simulink model "openWaterModel"  (R2020a)
settings: Solver=FixedStepAuto  StartTime=0.0  StopTime=inf  FixedStep=Ts  RelTol=1e-3  EnableMultiTasking=on
values from neighbouring files (symbols this model uses):
  ctrlMap =     [init_Kite.mat]
  Ts = 0.01    [init_Kite.mat]
undefined symbols (not defined in the file or in its folder): initializeBussesFromBlock, IO397, standard
libraries: xpcutilitieslib x172, hdlsllib x100, simulink x36, dspsigops x13, slrtlib x4, xpcseriallib x3, speedgoatlib_fpga_analog_io x2, xpcrtudplib x2, speedgoatlib_fpga_dio x1, speedgoatlib_fpga_quadrature x1, speedgoatlib_IO581 x1, speedgoatlib_fpga x1
(part 3 of 4)

== system openWaterModel/Sensor Processing/IMU Processing/Controller1/FilteredPIDController2 ==
  note: Tau with minimum
  note: Anti-winding
  del_u : Inport
  Abs : Abs
  Add1 : Sum  Inputs=+++
  Add2 : Sum  Inputs=+-
  Constant : Constant
  Constant1 : Constant  Value=0
  Constant2 : Constant
  Divide{1..4} (4 alike) : Product  Inputs=*/
  Int_reset : Constant  Value=0
  Integrator : Integrator
  Integrator3 : Integrator  ExternalReset=either
  Max : MinMax  Function=max  Inputs=2
  Product : Product
  Product1 : Product
  RollKd : Gain
  RollKi : Gain  Gain=0
  RollKp : Gain  Gain=3
  RollTau : Constant  Value=0.02
  Switch : Switch  Threshold=30
  Weighted Sample Time : SampleTimeMath  TsampMathOp=Ts Only
  const : Constant
  y : Outport
  wires:
  Product1/1 -> Divide2/1
  [stop_trig] -> Product1/1
  RollKi/1 -> Product1/2
  Switch/1 -> [stop_trig]
  Constant2/1 -> Switch/3
  Constant1/1 -> Switch/1
  Abs/1 -> Switch/2
  [y] -> Abs/1
  Add2/1 -> Integrator/1, Product/2
  Divide4/1 -> Add2/2
  del_u/1 -> Add2/1
  [Tau] -> Divide4/2
  [Tau] -> Divide3/2
  Divide3/1 -> Add1/3
  RollKp/1 -> Divide3/1
  Product/1 -> Add1/1
  Integrator3/1 -> Add1/2
  Divide2/1 -> Integrator3/1
  [Tau] -> Divide2/2
  Integrator/1 -> RollKi/1, Divide4/1, RollKp/1
  Divide1/1 -> Product/1
  [Tau] -> Divide1/2
  Constant/1 -> RollKd/1
  RollKd/1 -> Divide1/1
  Max/1 -> [Tau]
  Weighted Sample Time/1 -> Max/1
  const/1 -> Weighted Sample Time/1
  Add1/1 -> y/1, [y]
  RollTau/1 -> Max/2
  Int_reset/1 -> Integrator3/2

== system openWaterModel/Sensor Processing/IMU Processing/Controller1/FilteredPIDController_Pitchold ==
  del_u : Inport
  Add : Sum  Inputs=+-
  Add1 : Sum  Inputs=+++
  Divide : Product  Inputs=*/
  Integrator : Integrator
  Integrator1 : Integrator
  Integrator2 : Integrator
  Max : MinMax  Function=max  Inputs=2
  PitchKd : Gain
  PitchKi : Gain  Gain=0
  PitchKp : Gain
  PitchTau : Constant  Value=0.1
  Weighted Sample Time : SampleTimeMath  TsampMathOp=Ts Only
  const : Constant
  y : Outport
  wires:
  PitchTau/1 -> Max/2
  Divide/1 -> y/1, [y]
  Add/1 -> Integrator/1
  const/1 -> Weighted Sample Time/1
  Integrator/1 -> Add1/1
  Integrator1/1 -> Integrator2/1
  [y] -> Add/2
  Max/1 -> Divide/2
  PitchKd/1 -> Add1/3
  Add1/1 -> Divide/1
  PitchKi/1 -> Integrator1/1
  PitchKp/1 -> Add/1
  Weighted Sample Time/1 -> Max/1
  Integrator2/1 -> Add1/2
  del_u/1 -> PitchKd/1, PitchKi/1, PitchKp/1

== system openWaterModel/Sensor Processing/IMU Processing/Controller1/FilteredPIDController_oldRoll ==
  del_u : Inport
  Add : Sum  Inputs=+-
  Add1 : Sum  Inputs=+++
  Divide : Product  Inputs=*/
  Integrator : Integrator
  Integrator1 : Integrator
  Integrator2 : Integrator
  Max : MinMax  Function=max  Inputs=2
  RollKd : Gain
  RollKi : Gain  Gain=0
  RollKp : Gain
  RollTau : Constant  Value=0.1
  Weighted Sample Time : SampleTimeMath  TsampMathOp=Ts Only
  const : Constant
  y : Outport
  wires:
  RollTau/1 -> Max/2
  Divide/1 -> y/1, [y]
  Add/1 -> Integrator/1
  const/1 -> Weighted Sample Time/1
  Integrator/1 -> Add1/1
  Integrator1/1 -> Integrator2/1
  [y] -> Add/2
  Max/1 -> Divide/2
  RollKd/1 -> Add1/3
  Add1/1 -> Divide/1
  RollKi/1 -> Integrator1/1
  RollKp/1 -> Add/1
  Weighted Sample Time/1 -> Max/1
  Integrator2/1 -> Add1/2
  del_u/1 -> RollKd/1, RollKi/1, RollKp/1

== system openWaterModel/Sensor Processing/IMU Processing/Controller1/FilteredPIDController_oldYaw ==
  del_u : Inport
  Add : Sum  Inputs=+-
  Add1 : Sum  Inputs=+++
  Divide : Product  Inputs=*/
  Integrator : Integrator
  Integrator1 : Integrator
  Integrator2 : Integrator
  Max : MinMax  Function=max  Inputs=2
  Weighted Sample Time : SampleTimeMath  TsampMathOp=Ts Only
  YawKd : Gain  Gain=0.2
  YawKi : Gain  Gain=0.3
  YawKp : Gain  Gain=0.1
  YawTau : Constant  Value=0.4
  const : Constant
  y : Outport
  wires:
  YawTau/1 -> Max/2
  Divide/1 -> y/1, [y]
  Add/1 -> Integrator/1
  const/1 -> Weighted Sample Time/1
  Integrator/1 -> Add1/1
  Integrator1/1 -> Integrator2/1
  [y] -> Add/2
  Max/1 -> Divide/2
  YawKd/1 -> Add1/3
  Add1/1 -> Divide/1
  YawKi/1 -> Integrator1/1
  YawKp/1 -> Add/1
  Weighted Sample Time/1 -> Max/1
  Integrator2/1 -> Add1/2
  del_u/1 -> YawKd/1, YawKi/1, YawKp/1

== system openWaterModel/Sensor Processing/IMU Processing/Kite Measurements /Enabled Subsystem ==
  Double : Inport
  Enable : EnablePort
  Out1 : Outport
  wires:
  Double/1 -> Out1/1

== system openWaterModel/Sensor Processing/IMU Processing/Kite Measurements /Enabled Subsystem1 ==
  Double : Inport
  Enable : EnablePort
  Out1 : Outport
  wires:
  Double/1 -> Out1/1

== system openWaterModel/Sensor Processing/IMU Processing/Kite Measurements /Enabled Subsystem10 ==
  Double : Inport
  Enable : EnablePort
  Out1 : Outport
  wires:
  Double/1 -> Out1/1

== system openWaterModel/Sensor Processing/IMU Processing/Kite Measurements /Enabled Subsystem11 ==
  Double : Inport
  Enable : EnablePort
  Out1 : Outport
  wires:
  Double/1 -> Out1/1

== system openWaterModel/Sensor Processing/IMU Processing/Kite Measurements /Enabled Subsystem12 ==
  Double : Inport
  Enable : EnablePort
  Out1 : Outport
  wires:
  Double/1 -> Out1/1

== system openWaterModel/Sensor Processing/IMU Processing/Kite Measurements /Enabled Subsystem13 ==
  Double : Inport
  Enable : EnablePort
  Out1 : Outport
  wires:
  Double/1 -> Out1/1

== system openWaterModel/Sensor Processing/IMU Processing/Kite Measurements /Enabled Subsystem14 ==
  Double : Inport
  Enable : EnablePort
  Out1 : Outport
  wires:
  Double/1 -> Out1/1

== system openWaterModel/Sensor Processing/IMU Processing/Kite Measurements /Enabled Subsystem15 ==
  Double : Inport
  Enable : EnablePort
  Out1 : Outport
  wires:
  Double/1 -> Out1/1

== system openWaterModel/Sensor Processing/IMU Processing/Kite Measurements /Enabled Subsystem16 ==
  Double : Inport
  Enable : EnablePort
  Out1 : Outport
  wires:
  Double/1 -> Out1/1

== system openWaterModel/Sensor Processing/IMU Processing/Kite Measurements /Enabled Subsystem17 ==
  Double : Inport
  Enable : EnablePort
  Out1 : Outport
  wires:
  Double/1 -> Out1/1

== system openWaterModel/Sensor Processing/IMU Processing/Kite Measurements /Enabled Subsystem18 ==
  Double : Inport
  Enable : EnablePort
  Out1 : Outport
  wires:
  Double/1 -> Out1/1

== system openWaterModel/Sensor Processing/IMU Processing/Kite Measurements /Enabled Subsystem19 ==
  Double : Inport
  Enable : EnablePort
  Out1 : Outport
  wires:
  Double/1 -> Out1/1

== system openWaterModel/Sensor Processing/IMU Processing/Kite Measurements /Enabled Subsystem2 ==
  Double : Inport
  Enable : EnablePort
  Out1 : Outport
  wires:
  Double/1 -> Out1/1

== system openWaterModel/Sensor Processing/IMU Processing/Kite Measurements /Enabled Subsystem3 ==
  Double : Inport
  Enable : EnablePort
  Out1 : Outport
  wires:
  Double/1 -> Out1/1

== system openWaterModel/Sensor Processing/IMU Processing/Kite Measurements /Enabled Subsystem4 ==
  Double : Inport
  Enable : EnablePort
  Out1 : Outport
  wires:
  Double/1 -> Out1/1

== system openWaterModel/Sensor Processing/IMU Processing/Kite Measurements /Enabled Subsystem5 ==
  Double : Inport
  Enable : EnablePort
  Out1 : Outport
  wires:
  Double/1 -> Out1/1

== system openWaterModel/Sensor Processing/IMU Processing/Kite Measurements /Enabled Subsystem6 ==
  Double : Inport
  Enable : EnablePort
  Out1 : Outport
  wires:
  Double/1 -> Out1/1

== system openWaterModel/Sensor Processing/IMU Processing/Kite Measurements /Enabled Subsystem7 ==
  Double : Inport
  Enable : EnablePort
  Out1 : Outport
  wires:
  Double/1 -> Out1/1

== system openWaterModel/Sensor Processing/IMU Processing/Kite Measurements /Enabled Subsystem8 ==
  Double : Inport
  Enable : EnablePort
  Out1 : Outport
  wires:
  Double/1 -> Out1/1

== system openWaterModel/Sensor Processing/IMU Processing/Kite Measurements /Enabled Subsystem9 ==
  Double : Inport
  Enable : EnablePort
  Out1 : Outport
  wires:
  Double/1 -> Out1/1

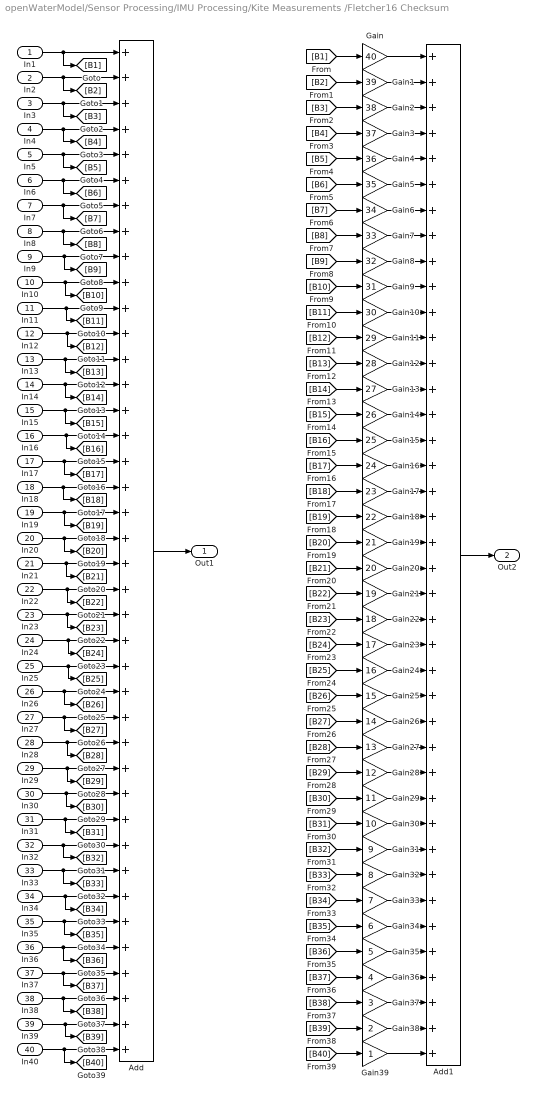
== system openWaterModel/Sensor Processing/IMU Processing/Kite Measurements /Fletcher16 Checksum ==
  In1 : Inport
  In2 : Inport  Port=2
  In3 : Inport  Port=3
  In4 : Inport  Port=4
  In5 : Inport  Port=5
  In6 : Inport  Port=6
  In7 : Inport  Port=7
  In8 : Inport  Port=8
  In9 : Inport  Port=9
  In10 : Inport  Port=10
  In11 : Inport  Port=11
  In12 : Inport  Port=12
  In13 : Inport  Port=13
  In14 : Inport  Port=14
  In15 : Inport  Port=15
  In16 : Inport  Port=16
  In17 : Inport  Port=17
  In18 : Inport  Port=18
  In19 : Inport  Port=19
  In20 : Inport  Port=20
  In21 : Inport  Port=21
  In22 : Inport  Port=22
  In23 : Inport  Port=23
  In24 : Inport  Port=24
  In25 : Inport  Port=25
  In26 : Inport  Port=26
  In27 : Inport  Port=27
  In28 : Inport  Port=28
  In29 : Inport  Port=29
  In30 : Inport  Port=30
  In31 : Inport  Port=31
  In32 : Inport  Port=32
  In33 : Inport  Port=33
  In34 : Inport  Port=34
  In35 : Inport  Port=35
  In36 : Inport  Port=36
  In37 : Inport  Port=37
  In38 : Inport  Port=38
  In39 : Inport  Port=39
  In40 : Inport  Port=40
  Add : Sum  Inputs=++++++++++++++++++++++++++++++++++++++++
  Add1 : Sum  Inputs=++++++++++++++++++++++++++++++++++++++++
  Gain : Gain  Gain=40  OutDataTypeStr=uint8
  Gain1 : Gain  Gain=39  OutDataTypeStr=uint8
  Gain10 : Gain  Gain=30  OutDataTypeStr=uint8
  Gain11 : Gain  Gain=29  OutDataTypeStr=uint8
  Gain12 : Gain  Gain=28  OutDataTypeStr=uint8
  Gain13 : Gain  Gain=27  OutDataTypeStr=uint8
  Gain14 : Gain  Gain=26  OutDataTypeStr=uint8
  Gain15 : Gain  Gain=25  OutDataTypeStr=uint8
  Gain16 : Gain  Gain=24  OutDataTypeStr=uint8
  Gain17 : Gain  Gain=23  OutDataTypeStr=uint8
  Gain18 : Gain  Gain=22  OutDataTypeStr=uint8
  Gain19 : Gain  Gain=21  OutDataTypeStr=uint8
  Gain2 : Gain  Gain=38  OutDataTypeStr=uint8
  Gain20 : Gain  Gain=20  OutDataTypeStr=uint8
  Gain21 : Gain  Gain=19  OutDataTypeStr=uint8
  Gain22 : Gain  Gain=18  OutDataTypeStr=uint8
  Gain23 : Gain  Gain=17  OutDataTypeStr=uint8
  Gain24 : Gain  Gain=16  OutDataTypeStr=uint8
  Gain25 : Gain  Gain=15  OutDataTypeStr=uint8
  Gain26 : Gain  Gain=14  OutDataTypeStr=uint8
  Gain27 : Gain  Gain=13  OutDataTypeStr=uint8
  Gain28 : Gain  Gain=12  OutDataTypeStr=uint8
  Gain29 : Gain  Gain=11  OutDataTypeStr=uint8
  Gain3 : Gain  Gain=37  OutDataTypeStr=uint8
  Gain30 : Gain  Gain=10  OutDataTypeStr=uint8
  Gain31 : Gain  Gain=9  OutDataTypeStr=uint8
  Gain32 : Gain  Gain=8  OutDataTypeStr=uint8
  Gain33 : Gain  Gain=7  OutDataTypeStr=uint8
  Gain34 : Gain  Gain=6  OutDataTypeStr=uint8
  Gain35 : Gain  Gain=5  OutDataTypeStr=uint8
  Gain36 : Gain  Gain=4  OutDataTypeStr=uint8
  Gain37 : Gain  Gain=3  OutDataTypeStr=uint8
  Gain38 : Gain  Gain=2  OutDataTypeStr=uint8
  Gain39 : Gain  OutDataTypeStr=uint8
  Gain4 : Gain  Gain=36  OutDataTypeStr=uint8
  Gain5 : Gain  Gain=35  OutDataTypeStr=uint8
  Gain6 : Gain  Gain=34  OutDataTypeStr=uint8
  Gain7 : Gain  Gain=33  OutDataTypeStr=uint8
  Gain8 : Gain  Gain=32  OutDataTypeStr=uint8
  Gain9 : Gain  Gain=31  OutDataTypeStr=uint8
  Out1 : Outport
  Out2 : Outport  Port=2
  wires:
  In3/1 -> [B3], Add/3
  [B4] -> Gain3/1
  In2/1 -> [B2], Add/2
  [B1] -> Gain/1
  Add1/1 -> Out2/1
  In4/1 -> [B4], Add/4
  [B3] -> Gain2/1
  In6/1 -> [B6], Add/6
  In5/1 -> [B5], Add/5
  [B2] -> Gain1/1
  [B5] -> Gain4/1
  In1/1 -> Add/1, [B1]
  Add/1 -> Out1/1
  In7/1 -> [B7], Add/7
  In8/1 -> [B8], Add/8
  In9/1 -> [B9], Add/9
  In10/1 -> [B10], Add/10
  In11/1 -> [B11], Add/11
  In12/1 -> [B12], Add/12
  In13/1 -> [B13], Add/13
  In14/1 -> [B14], Add/14
  In15/1 -> [B15], Add/15
  In16/1 -> [B16], Add/16
  In17/1 -> [B17], Add/17
  In18/1 -> [B18], Add/18
  In19/1 -> [B19], Add/19
  In20/1 -> [B20], Add/20
  In21/1 -> [B21], Add/21
  In22/1 -> [B22], Add/22
  In23/1 -> [B23], Add/23
  In24/1 -> [B24], Add/24
  In25/1 -> [B25], Add/25
  In26/1 -> [B26], Add/26
  In27/1 -> [B27], Add/27
  In28/1 -> [B28], Add/28
  In29/1 -> [B29], Add/29
  In30/1 -> [B30], Add/30
  In31/1 -> [B31], Add/31
  In32/1 -> [B32], Add/32
  In33/1 -> [B33], Add/33
  In34/1 -> [B34], Add/34
  In35/1 -> [B35], Add/35
  In36/1 -> [B36], Add/36
  In37/1 -> [B37], Add/37
  In38/1 -> [B38], Add/38
  In39/1 -> [B39], Add/39
  In40/1 -> [B40], Add/40
  Gain/1 -> Add1/1
  Gain1/1 -> Add1/2
  Gain2/1 -> Add1/3
  Gain3/1 -> Add1/4
  Gain4/1 -> Add1/5
  [B6] -> Gain5/1
  Gain5/1 -> Add1/6
  [B7] -> Gain6/1
  Gain6/1 -> Add1/7
  Gain7/1 -> Add1/8
  [B8] -> Gain7/1
  [B9] -> Gain8/1
  Gain8/1 -> Add1/9
  Gain9/1 -> Add1/10
  [B10] -> Gain9/1
  [B11] -> Gain10/1
  Gain10/1 -> Add1/11
  [B12] -> Gain11/1
  [B13] -> Gain12/1
  [B14] -> Gain13/1
  Gain13/1 -> Add1/14
  [B15] -> Gain14/1
  Gain14/1 -> Add1/15
  [B16] -> Gain15/1
  Gain15/1 -> Add1/16
  [B17] -> Gain16/1
  Gain16/1 -> Add1/17
  [B18] -> Gain17/1
  Gain17/1 -> Add1/18
  [B19] -> Gain18/1
  Gain18/1 -> Add1/19
  [B20] -> Gain19/1
  Gain19/1 -> Add1/20
  [B21] -> Gain20/1
  Gain20/1 -> Add1/21
  [B22] -> Gain21/1
  Gain21/1 -> Add1/22
  [B23] -> Gain22/1
  Gain22/1 -> Add1/23
  [B24] -> Gain23/1
  Gain23/1 -> Add1/24
  [B25] -> Gain24/1
  Gain24/1 -> Add1/25
  [B26] -> Gain25/1
  Gain25/1 -> Add1/26
  [B27] -> Gain26/1
  Gain26/1 -> Add1/27
  [B28] -> Gain27/1
  Gain27/1 -> Add1/28
  [B29] -> Gain28/1
  Gain28/1 -> Add1/29
  [B30] -> Gain29/1
  Gain29/1 -> Add1/30
  [B31] -> Gain30/1
  Gain30/1 -> Add1/31
  [B32] -> Gain31/1
  Gain31/1 -> Add1/32
  [B33] -> Gain32/1
  Gain32/1 -> Add1/33
  [B34] -> Gain33/1
  Gain33/1 -> Add1/34
  [B35] -> Gain34/1
  Gain34/1 -> Add1/35
  [B36] -> Gain35/1
  Gain35/1 -> Add1/36
  [B37] -> Gain36/1
  Gain36/1 -> Add1/37
  [B38] -> Gain37/1
  Gain37/1 -> Add1/38
  [B39] -> Gain38/1
  Gain38/1 -> Add1/39
  [B40] -> Gain39/1
  Gain39/1 -> Add1/40
  Gain11/1 -> Add1/12
  Gain12/1 -> Add1/13

== system openWaterModel/Sensor Processing/IMU Processing/Kite Measurements /Fletcher16 Checksum1 ==
  In1 : Inport
  In2 : Inport  Port=2
  In3 : Inport  Port=3
  In4 : Inport  Port=4
  Add : Sum  Inputs=4
  Add1 : Sum  Inputs=++++
  Gain : Gain  Gain=4  OutDataTypeStr=uint8
  Gain1 : Gain  Gain=3  OutDataTypeStr=uint8
  Gain2 : Gain  Gain=2  OutDataTypeStr=uint8
  Gain3 : Gain  OutDataTypeStr=uint8
  Out1 : Outport
  Out2 : Outport  Port=2
  wires:
  Gain3/1 -> Add1/4
  Gain2/1 -> Add1/3
  Gain1/1 -> Add1/2
  Gain/1 -> Add1/1
  Add/1 -> Out1/1
  In1/1 -> [B1], Add/1
  [B2] -> Gain1/1
  [B3] -> Gain2/1
  In4/1 -> [B4], Add/4
  Add1/1 -> Out2/1
  [B1] -> Gain/1
  In2/1 -> [B2], Add/2
  [B4] -> Gain3/1
  In3/1 -> [B3], Add/3

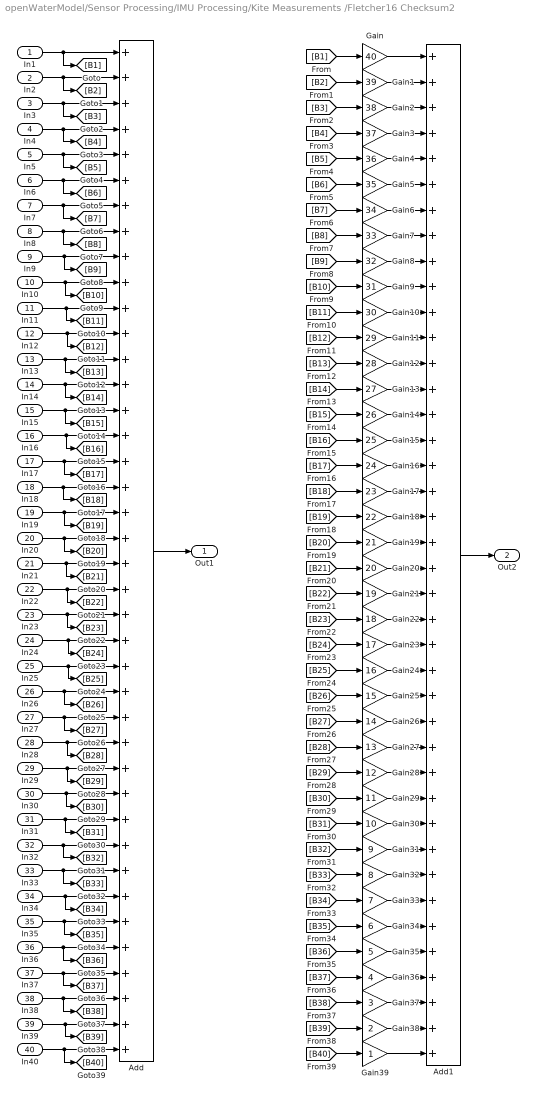
== system openWaterModel/Sensor Processing/IMU Processing/Kite Measurements /Fletcher16 Checksum2 ==
  In1 : Inport
  In2 : Inport  Port=2
  In3 : Inport  Port=3
  In4 : Inport  Port=4
  In5 : Inport  Port=5
  In6 : Inport  Port=6
  In7 : Inport  Port=7
  In8 : Inport  Port=8
  In9 : Inport  Port=9
  In10 : Inport  Port=10
  In11 : Inport  Port=11
  In12 : Inport  Port=12
  In13 : Inport  Port=13
  In14 : Inport  Port=14
  In15 : Inport  Port=15
  In16 : Inport  Port=16
  In17 : Inport  Port=17
  In18 : Inport  Port=18
  In19 : Inport  Port=19
  In20 : Inport  Port=20
  In21 : Inport  Port=21
  In22 : Inport  Port=22
  In23 : Inport  Port=23
  In24 : Inport  Port=24
  In25 : Inport  Port=25
  In26 : Inport  Port=26
  In27 : Inport  Port=27
  In28 : Inport  Port=28
  In29 : Inport  Port=29
  In30 : Inport  Port=30
  In31 : Inport  Port=31
  In32 : Inport  Port=32
  In33 : Inport  Port=33
  In34 : Inport  Port=34
  In35 : Inport  Port=35
  In36 : Inport  Port=36
  In37 : Inport  Port=37
  In38 : Inport  Port=38
  In39 : Inport  Port=39
  In40 : Inport  Port=40
  Add : Sum  Inputs=++++++++++++++++++++++++++++++++++++++++
  Add1 : Sum  Inputs=++++++++++++++++++++++++++++++++++++++++
  Gain : Gain  Gain=40  OutDataTypeStr=uint8
  Gain1 : Gain  Gain=39  OutDataTypeStr=uint8
  Gain10 : Gain  Gain=30  OutDataTypeStr=uint8
  Gain11 : Gain  Gain=29  OutDataTypeStr=uint8
  Gain12 : Gain  Gain=28  OutDataTypeStr=uint8
  Gain13 : Gain  Gain=27  OutDataTypeStr=uint8
  Gain14 : Gain  Gain=26  OutDataTypeStr=uint8
  Gain15 : Gain  Gain=25  OutDataTypeStr=uint8
  Gain16 : Gain  Gain=24  OutDataTypeStr=uint8
  Gain17 : Gain  Gain=23  OutDataTypeStr=uint8
  Gain18 : Gain  Gain=22  OutDataTypeStr=uint8
  Gain19 : Gain  Gain=21  OutDataTypeStr=uint8
  Gain2 : Gain  Gain=38  OutDataTypeStr=uint8
  Gain20 : Gain  Gain=20  OutDataTypeStr=uint8
  Gain21 : Gain  Gain=19  OutDataTypeStr=uint8
  Gain22 : Gain  Gain=18  OutDataTypeStr=uint8
  Gain23 : Gain  Gain=17  OutDataTypeStr=uint8
  Gain24 : Gain  Gain=16  OutDataTypeStr=uint8
  Gain25 : Gain  Gain=15  OutDataTypeStr=uint8
  Gain26 : Gain  Gain=14  OutDataTypeStr=uint8
  Gain27 : Gain  Gain=13  OutDataTypeStr=uint8
  Gain28 : Gain  Gain=12  OutDataTypeStr=uint8
  Gain29 : Gain  Gain=11  OutDataTypeStr=uint8
  Gain3 : Gain  Gain=37  OutDataTypeStr=uint8
  Gain30 : Gain  Gain=10  OutDataTypeStr=uint8
  Gain31 : Gain  Gain=9  OutDataTypeStr=uint8
  Gain32 : Gain  Gain=8  OutDataTypeStr=uint8
  Gain33 : Gain  Gain=7  OutDataTypeStr=uint8
  Gain34 : Gain  Gain=6  OutDataTypeStr=uint8
  Gain35 : Gain  Gain=5  OutDataTypeStr=uint8
  Gain36 : Gain  Gain=4  OutDataTypeStr=uint8
  Gain37 : Gain  Gain=3  OutDataTypeStr=uint8
  Gain38 : Gain  Gain=2  OutDataTypeStr=uint8
  Gain39 : Gain  OutDataTypeStr=uint8
  Gain4 : Gain  Gain=36  OutDataTypeStr=uint8
  Gain5 : Gain  Gain=35  OutDataTypeStr=uint8
  Gain6 : Gain  Gain=34  OutDataTypeStr=uint8
  Gain7 : Gain  Gain=33  OutDataTypeStr=uint8
  Gain8 : Gain  Gain=32  OutDataTypeStr=uint8
  Gain9 : Gain  Gain=31  OutDataTypeStr=uint8
  Out1 : Outport
  Out2 : Outport  Port=2
  wires:
  In3/1 -> [B3], Add/3
  [B4] -> Gain3/1
  In2/1 -> [B2], Add/2
  [B1] -> Gain/1
  Add1/1 -> Out2/1
  In4/1 -> [B4], Add/4
  [B3] -> Gain2/1
  In6/1 -> [B6], Add/6
  In5/1 -> [B5], Add/5
  [B2] -> Gain1/1
  [B5] -> Gain4/1
  In1/1 -> Add/1, [B1]
  Add/1 -> Out1/1
  In7/1 -> [B7], Add/7
  In8/1 -> [B8], Add/8
  In9/1 -> [B9], Add/9
  In10/1 -> [B10], Add/10
  In11/1 -> [B11], Add/11
  In12/1 -> [B12], Add/12
  In13/1 -> [B13], Add/13
  In14/1 -> [B14], Add/14
  In15/1 -> [B15], Add/15
  In16/1 -> [B16], Add/16
  In17/1 -> [B17], Add/17
  In18/1 -> [B18], Add/18
  In19/1 -> [B19], Add/19
  In20/1 -> [B20], Add/20
  In21/1 -> [B21], Add/21
  In22/1 -> [B22], Add/22
  In23/1 -> [B23], Add/23
  In24/1 -> [B24], Add/24
  In25/1 -> [B25], Add/25
  In26/1 -> [B26], Add/26
  In27/1 -> [B27], Add/27
  In28/1 -> [B28], Add/28
  In29/1 -> [B29], Add/29
  In30/1 -> [B30], Add/30
  In31/1 -> [B31], Add/31
  In32/1 -> [B32], Add/32
  In33/1 -> [B33], Add/33
  In34/1 -> [B34], Add/34
  In35/1 -> [B35], Add/35
  In36/1 -> [B36], Add/36
  In37/1 -> [B37], Add/37
  In38/1 -> [B38], Add/38
  In39/1 -> [B39], Add/39
  In40/1 -> [B40], Add/40
  Gain/1 -> Add1/1
  Gain1/1 -> Add1/2
  Gain2/1 -> Add1/3
  Gain3/1 -> Add1/4
  Gain4/1 -> Add1/5
  [B6] -> Gain5/1
  Gain5/1 -> Add1/6
  [B7] -> Gain6/1
  Gain6/1 -> Add1/7
  Gain7/1 -> Add1/8
  [B8] -> Gain7/1
  [B9] -> Gain8/1
  Gain8/1 -> Add1/9
  Gain9/1 -> Add1/10
  [B10] -> Gain9/1
  [B11] -> Gain10/1
  Gain10/1 -> Add1/11
  [B12] -> Gain11/1
  [B13] -> Gain12/1
  [B14] -> Gain13/1
  Gain13/1 -> Add1/14
  [B15] -> Gain14/1
  Gain14/1 -> Add1/15
  [B16] -> Gain15/1
  Gain15/1 -> Add1/16
  [B17] -> Gain16/1
  Gain16/1 -> Add1/17
  [B18] -> Gain17/1
  Gain17/1 -> Add1/18
  [B19] -> Gain18/1
  Gain18/1 -> Add1/19
  [B20] -> Gain19/1
  Gain19/1 -> Add1/20
  [B21] -> Gain20/1
  Gain20/1 -> Add1/21
  [B22] -> Gain21/1
  Gain21/1 -> Add1/22
  [B23] -> Gain22/1
  Gain22/1 -> Add1/23
  [B24] -> Gain23/1
  Gain23/1 -> Add1/24
  [B25] -> Gain24/1
  Gain24/1 -> Add1/25
  [B26] -> Gain25/1
  Gain25/1 -> Add1/26
  [B27] -> Gain26/1
  Gain26/1 -> Add1/27
  [B28] -> Gain27/1
  Gain27/1 -> Add1/28
  [B29] -> Gain28/1
  Gain28/1 -> Add1/29
  [B30] -> Gain29/1
  Gain29/1 -> Add1/30
  [B31] -> Gain30/1
  Gain30/1 -> Add1/31
  [B32] -> Gain31/1
  Gain31/1 -> Add1/32
  [B33] -> Gain32/1
  Gain32/1 -> Add1/33
  [B34] -> Gain33/1
  Gain33/1 -> Add1/34
  [B35] -> Gain34/1
  Gain34/1 -> Add1/35
  [B36] -> Gain35/1
  Gain35/1 -> Add1/36
  [B37] -> Gain36/1
  Gain36/1 -> Add1/37
  [B38] -> Gain37/1
  Gain37/1 -> Add1/38
  [B39] -> Gain38/1
  Gain38/1 -> Add1/39
  [B40] -> Gain39/1
  Gain39/1 -> Add1/40
  Gain11/1 -> Add1/12
  Gain12/1 -> Add1/13

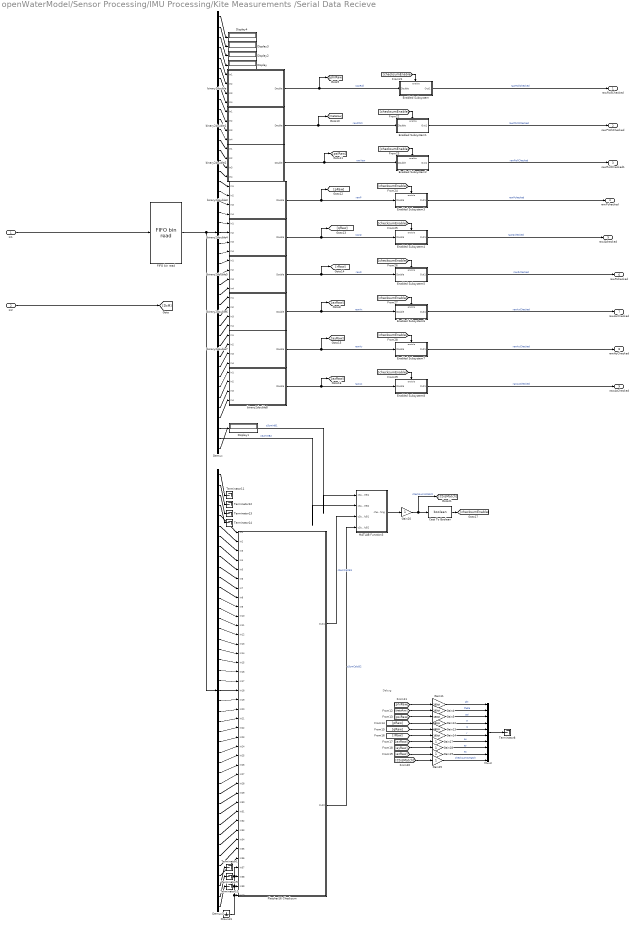
== system openWaterModel/Sensor Processing/IMU Processing/Kite Measurements /Serial Data Recieve ==
  note: Debug
  In1 : Inport
  In2 : Inport  Port=2
  Cast To Boolean : DataTypeConversion  OutDataTypeStr=boolean
  Demux : Demux  Outputs=43
  Demux3 : Demux  Outputs=43
  Display{,1..4} (5 alike) : Display
      Display settings: Format=hex (Stored Integer)
      Display2 settings: Format=hex (Stored Integer)
      Display3 settings: Format=hex (Stored Integer)
      Display4 settings: Format=hex (Stored Integer)
  Enabled Subsystem : Subsystem  TreatAsAtomicUnit=on
  Enabled Subsystem1 : Subsystem  TreatAsAtomicUnit=on
  Enabled Subsystem2 : Subsystem  TreatAsAtomicUnit=on
  Enabled Subsystem3 : Subsystem  TreatAsAtomicUnit=on
  Enabled Subsystem4 : Subsystem  TreatAsAtomicUnit=on
  Enabled Subsystem5 : Subsystem  TreatAsAtomicUnit=on
  Enabled Subsystem6 : Subsystem  TreatAsAtomicUnit=on
  Enabled Subsystem7 : Subsystem  TreatAsAtomicUnit=on
  Enabled Subsystem8 : Subsystem  TreatAsAtomicUnit=on
  "FIFO bin read " : xpcseriallib/FIFO bin read   header={[0x47 0xBB 0x3C 0x2B]}  lengths=[42]  hold=Hold last output if no new data  enable=off  maxsize=42  outputtype=8 bit uint null terminated  sampletime=0.01
      settings: SourceProductBaseCode=XP
  Fletcher16 Checksum : Subsystem
  Gain{4..5,11..14} (6 alike) : Gain  Gain=180/pi
  Gain{17..20,25} (5 alike) : Gain
  Ground1 : Ground
  MATLAB Function3 : MATLAB Function  TreatAsAtomicUnit=on
  Mux3 : Mux  Inputs=10
  Terminator{1,8..14} (8 alike) : Terminator
  binary2double : Subsystem
  binary2double1 : Subsystem
  binary2double2 : Subsystem
  binary2double3 : Subsystem
  binary2double4 : Subsystem
  binary2double5 : Subsystem
  binary2double6 : Subsystem
  binary2double7 : Subsystem
  binary2double8 : Subsystem
  rawRollChecked : Outport
  rawPitchChecked : Outport  Port=2
  rawRollChecked1 : Outport  Port=3
  rawPchecked : Outport  Port=4
  rawQchecked : Outport  Port=5
  rawRchecked : Outport  Port=6
  rawAxChecked : Outport  Port=7
  rawAyChecked : Outport  Port=8
  rawAzChecked : Outport  Port=9
  wires:
  Demux/29 -> binary2double6/1(In1)
  Gain5/1 -> Mux3/3  "psi"
  Demux/33 -> binary2double7/1(In1)
  Demux/16 -> binary2double2/4(In4)
  Demux3/37 -> Fletcher16 Checksum/33(In33)
  Demux/1 -> Display4/1
  Demux/10 -> binary2double1/2(In2)
  Demux/28 -> binary2double5/4(In4)
  binary2double6/1(Double) -> [axRaw], Enabled Subsystem6/1(Double)  "rawAx"
  [rRaw] -> Gain14/1
  Demux/7 -> binary2double/3(In3)
  MATLAB Function3/1(checksumIsMatching) -> Gain20/1
  Demux/17 -> binary2double3/1(In1)
  Demux/15 -> binary2double2/3(In3)
  Demux/27 -> binary2double5/3(In3)
  Fletcher16 Checksum/1(Out1) -> MATLAB Function3/3(cSumCalcB1)  "cSumCalcB1"
  Demux3/27 -> Fletcher16 Checksum/23(In23)
  Demux3/20 -> Fletcher16 Checksum/16(In16)
  Demux3/21 -> Fletcher16 Checksum/17(In17)
  Demux/5 -> binary2double/1(In1)
  Gain25/1 -> Mux3/10  "checksumIsMatch"
  Demux/21 -> binary2double4/1(In1)
  Demux/13 -> binary2double2/1(In1)
  Demux3/24 -> Fletcher16 Checksum/20(In20)
  Demux3/38 -> Fletcher16 Checksum/34(In34)
  Enabled Subsystem2/1(Out1) -> rawRollChecked1/1  "rawRollChecked"
  Demux/2 -> Display3/1
  Demux3/5 -> Fletcher16 Checksum/1(In1)
  Demux3/10 -> Fletcher16 Checksum/6(In6)
  Demux/37 -> binary2double8/1(In1)
  Demux/38 -> binary2double8/2(In2)
  [thetaRaw] -> Gain4/1
  [phiRaw] -> Gain11/1
  Demux3/18 -> Fletcher16 Checksum/14(In14)
  Demux/18 -> binary2double3/2(In2)
  Demux3/11 -> Fletcher16 Checksum/7(In7)
  Demux3/7 -> Fletcher16 Checksum/3(In3)
  Demux3/36 -> Fletcher16 Checksum/32(In32)
  [checksumEnable] -> Enabled Subsystem/Enable
  Demux/9 -> binary2double1/1(In1)
  Demux3/30 -> Fletcher16 Checksum/26(In26)
  Demux/26 -> binary2double5/2(In2)
  binary2double7/1(Double) -> Enabled Subsystem7/1(Double), [ayRaw]  "rawAy"
  Demux3/13 -> Fletcher16 Checksum/9(In9)
  Gain19/1 -> Mux3/9  "az"
  Demux/3 -> Display2/1
  Gain18/1 -> Mux3/8  "ay"
  Demux/43 -> Display1/1
  [azRaw] -> Gain19/1
  Gain4/1 -> Mux3/2  "theta"
  binary2double1/1(Double) -> Enabled Subsystem1/1(Double), [thetaRaw]  "rawPitch"
  binary2double4/1(Double) -> Enabled Subsystem4/1(Double), [qRaw]  "rawQ"
  Demux3/40 -> Fletcher16 Checksum/36(In36)
  Demux3/14 -> Fletcher16 Checksum/10(In10)
  [checksumEnable] -> Enabled Subsystem8/Enable
  Demux3/17 -> Fletcher16 Checksum/13(In13)
  Demux3/9 -> Fletcher16 Checksum/5(In5)
  Demux/35 -> binary2double7/3(In3)
  Demux/31 -> binary2double6/3(In3)
  Gain12/1 -> Mux3/4  "p"
  Demux3/16 -> Fletcher16 Checksum/12(In12)
  Demux3/33 -> Fletcher16 Checksum/29(In29)
  Demux/24 -> binary2double4/4(In4)
  Demux3/15 -> Fletcher16 Checksum/11(In11)
  Demux3/19 -> Fletcher16 Checksum/15(In15)
  [checksumEnable] -> Enabled Subsystem7/Enable
  Demux3/31 -> Fletcher16 Checksum/27(In27)
  Demux3/26 -> Fletcher16 Checksum/22(In22)
  Demux3/29 -> Fletcher16 Checksum/25(In25)
  Demux3/22 -> Fletcher16 Checksum/18(In18)
  Demux3/2 -> Terminator12/1
  Enabled Subsystem4/1(Out1) -> rawQchecked/1  "rawQchecked"
  Gain20/1 -> [CSisMatch], Cast To Boolean/1  "checksumIsMatch"
  Demux3/35 -> Fletcher16 Checksum/31(In31)
  Demux/39 -> binary2double8/3(In3)
  binary2double5/1(Double) -> [rRaw], Enabled Subsystem5/1(Double)  "rawR"
  [pRaw] -> Gain12/1
  Demux3/1 -> Terminator11/1
  [axRaw] -> Gain17/1
  Demux3/34 -> Fletcher16 Checksum/30(In30)
  Demux/32 -> binary2double6/4(In4)
  binary2double/1(Double) -> Enabled Subsystem/1(Double), [phiRaw]  "rawRoll"
  Demux3/23 -> Fletcher16 Checksum/19(In19)
  Demux/6 -> binary2double/2(In2)
  [ayRaw] -> Gain18/1
  Gain11/1 -> Mux3/1  "phi"
  Demux3/3 -> Terminator13/1
  Demux/8 -> binary2double/4(In4)
  binary2double2/1(Double) -> Enabled Subsystem2/1(Double), [psiRaw]  "rawYaw"
  [qRaw] -> Gain13/1
  Enabled Subsystem/1(Out1) -> rawRollChecked/1  "rawRollChecked"
  [checksumEnable] -> Enabled Subsystem4/Enable
  Demux/14 -> binary2double2/2(In2)
  Demux/40 -> binary2double8/4(In4)
  [checksumEnable] -> Enabled Subsystem6/Enable
  "FIFO bin read "/1 -> Demux3/1, Demux/1
  Gain13/1 -> Mux3/5  "q"
  Demux/34 -> binary2double7/2(In2)
  [checksumEnable] -> Enabled Subsystem1/Enable
  Demux/25 -> binary2double5/1(In1)
  Demux/36 -> binary2double7/4(In4)
  binary2double8/1(Double) -> Enabled Subsystem8/1(Double), [azRaw]  "rawAz"
  Demux3/42 -> Terminator9/1
  binary2double3/1(Double) -> Enabled Subsystem3/1(Double), [pRaw]  "rawP"
  Ground1/1 -> Fletcher16 Checksum/37(In37), Fletcher16 Checksum/38(In38), Fletcher16 Checksum/39(In39), Fletcher16 Checksum/40(In40)
  Demux3/28 -> Fletcher16 Checksum/24(In24)
  Gain14/1 -> Mux3/6  "r"
  Demux3/43 -> Terminator10/1
  [checksumEnable] -> Enabled Subsystem3/Enable
  [CSisMatch] -> Gain25/1
  Demux/41 -> MATLAB Function3/1(cSumInB1)  "cSumInB1"
  Cast To Boolean/1 -> [checksumEnable]
  Demux/11 -> binary2double1/3(In3)
  Demux3/39 -> Fletcher16 Checksum/35(In35)
  [checksumEnable] -> Enabled Subsystem2/Enable
  Demux/19 -> binary2double3/3(In3)
  Demux3/8 -> Fletcher16 Checksum/4(In4)
  Demux3/25 -> Fletcher16 Checksum/21(In21)
  Demux3/32 -> Fletcher16 Checksum/28(In28)
  Gain17/1 -> Mux3/7  "ax"
  Demux/20 -> binary2double3/4(In4)
  Demux3/6 -> Fletcher16 Checksum/2(In2)
  Demux/30 -> binary2double6/2(In2)
  Demux/42 -> MATLAB Function3/2(cSumInB2)  "cSumInB2"
  Demux/4 -> Display/1
  [psiRaw] -> Gain5/1
  Demux3/4 -> Terminator14/1
  [checksumEnable] -> Enabled Subsystem5/Enable
  Demux/22 -> binary2double4/2(In2)
  In1/1 -> "FIFO bin read "/1
  Demux/12 -> binary2double1/4(In4)
  Fletcher16 Checksum/2(Out2) -> MATLAB Function3/4(cSumCalcB2)  "cSumCalcB2"
  Enabled Subsystem6/1(Out1) -> rawAxChecked/1  "rawAxChecked"
  Demux/23 -> binary2double4/3(In3)
  Demux3/41 -> Terminator1/1
  Demux3/12 -> Fletcher16 Checksum/8(In8)
  Mux3/1 -> Terminator8/1
  In2/1 -> [DcM]
  Enabled Subsystem7/1(Out1) -> rawAyChecked/1  "rawAyChecked"
  Enabled Subsystem8/1(Out1) -> rawAzChecked/1  "rawAzChecked"
  Enabled Subsystem3/1(Out1) -> rawPchecked/1  "rawPchecked"
  Enabled Subsystem5/1(Out1) -> rawRchecked/1  "rawRchecked"
  Enabled Subsystem1/1(Out1) -> rawPitchChecked/1  "rawPitchChecked"

== system openWaterModel/Sensor Processing/IMU Processing/Kite Measurements /binary2double ==
  In1 : Inport
  In2 : Inport  Port=2
  In3 : Inport  Port=3
  In4 : Inport  Port=4
  Bit Packing {,1..4} (5 alike) : xpcutilitieslib/Bit Packing 
      settings: SourceProductBaseCode=XP
  Bit Shift1 : hdlsllib/Logic and Bit Operations/Bit Shift  mode=Shift Left Logical  N=16
  Bit Shift2 : hdlsllib/Logic and Bit Operations/Bit Shift  mode=Shift Left Logical  N=24
  Bit Shift3 : hdlsllib/Logic and Bit Operations/Bit Shift  mode=Shift Left Logical  N=8
  Bitwise Operator : simulink/Logic and Bit Operations/Bitwise Operator  logicop=OR  UseBitMask=off  NumInputPorts=4  BitMask=bin2dec('00000000')  BitMaskRealWorld=Stored Integer
  Cast To Double1 : DataTypeConversion  OutDataTypeStr=double
  Display{3,5..7,10..14} (9 alike) : Display
      settings: Format=hex (Stored Integer)
  Double : Outport
  wires:
  Bit Shift1/1 -> Bitwise Operator/2, Display10/1
  Bitwise Operator/1 -> Display14/1, "Bit Packing "/1
  Bit Packing 1/1 -> Bit Shift2/1
  Bit Packing 4/1 -> Bitwise Operator/4, Display13/1
  In1/1 -> Bit Packing 1/1, Display3/1
  In3/1 -> Bit Packing 3/1, Display6/1
  Bit Shift2/1 -> Bitwise Operator/1, Display11/1
  Bit Packing 2/1 -> Bit Shift1/1
  "Bit Packing "/1 -> Cast To Double1/1
  Bit Shift3/1 -> Bitwise Operator/3, Display12/1
  Bit Packing 3/1 -> Bit Shift3/1
  In2/1 -> Bit Packing 2/1, Display5/1
  In4/1 -> Bit Packing 4/1, Display7/1
  Cast To Double1/1 -> Double/1

== system openWaterModel/Sensor Processing/IMU Processing/Kite Measurements /binary2double1 ==
  In1 : Inport
  In2 : Inport  Port=2
  In3 : Inport  Port=3
  In4 : Inport  Port=4
  Bit Packing {,1..4} (5 alike) : xpcutilitieslib/Bit Packing 
      settings: SourceProductBaseCode=XP
  Bit Shift1 : hdlsllib/Logic and Bit Operations/Bit Shift  mode=Shift Left Logical  N=16
  Bit Shift2 : hdlsllib/Logic and Bit Operations/Bit Shift  mode=Shift Left Logical  N=24
  Bit Shift3 : hdlsllib/Logic and Bit Operations/Bit Shift  mode=Shift Left Logical  N=8
  Bitwise Operator : simulink/Logic and Bit Operations/Bitwise Operator  logicop=OR  UseBitMask=off  NumInputPorts=4  BitMask=bin2dec('00000000')  BitMaskRealWorld=Stored Integer
  Cast To Double1 : DataTypeConversion  OutDataTypeStr=double
  Display{3,5..7,10..14} (9 alike) : Display
      settings: Format=hex (Stored Integer)
  Double : Outport
  wires:
  Bit Shift1/1 -> Bitwise Operator/2, Display10/1
  Bitwise Operator/1 -> Display14/1, "Bit Packing "/1
  Bit Packing 1/1 -> Bit Shift2/1
  Bit Packing 4/1 -> Bitwise Operator/4, Display13/1
  In1/1 -> Bit Packing 1/1, Display3/1
  In3/1 -> Bit Packing 3/1, Display6/1
  Bit Shift2/1 -> Bitwise Operator/1, Display11/1
  Bit Packing 2/1 -> Bit Shift1/1
  "Bit Packing "/1 -> Cast To Double1/1
  Bit Shift3/1 -> Bitwise Operator/3, Display12/1
  Bit Packing 3/1 -> Bit Shift3/1
  In2/1 -> Bit Packing 2/1, Display5/1
  In4/1 -> Bit Packing 4/1, Display7/1
  Cast To Double1/1 -> Double/1

== system openWaterModel/Sensor Processing/IMU Processing/Kite Measurements /binary2double10 ==
  In1 : Inport
  In2 : Inport  Port=2
  In3 : Inport  Port=3
  In4 : Inport  Port=4
  Bit Packing {,1..4} (5 alike) : xpcutilitieslib/Bit Packing 
      settings: SourceProductBaseCode=XP
  Bit Shift1 : hdlsllib/Logic and Bit Operations/Bit Shift  mode=Shift Left Logical  N=16
  Bit Shift2 : hdlsllib/Logic and Bit Operations/Bit Shift  mode=Shift Left Logical  N=24
  Bit Shift3 : hdlsllib/Logic and Bit Operations/Bit Shift  mode=Shift Left Logical  N=8
  Bitwise Operator : simulink/Logic and Bit Operations/Bitwise Operator  logicop=OR  UseBitMask=off  NumInputPorts=4  BitMask=bin2dec('00000000')  BitMaskRealWorld=Stored Integer
  Cast To Double1 : DataTypeConversion  OutDataTypeStr=double
  Display{3,5..7,10..14} (9 alike) : Display
      settings: Format=hex (Stored Integer)
  Double : Outport
  wires:
  Bit Shift1/1 -> Bitwise Operator/2, Display10/1
  Bitwise Operator/1 -> Display14/1, "Bit Packing "/1
  Bit Packing 1/1 -> Bit Shift2/1
  Bit Packing 4/1 -> Bitwise Operator/4, Display13/1
  In1/1 -> Bit Packing 1/1, Display3/1
  In3/1 -> Bit Packing 3/1, Display6/1
  Bit Shift2/1 -> Bitwise Operator/1, Display11/1
  Bit Packing 2/1 -> Bit Shift1/1
  "Bit Packing "/1 -> Cast To Double1/1
  Bit Shift3/1 -> Bitwise Operator/3, Display12/1
  Bit Packing 3/1 -> Bit Shift3/1
  In2/1 -> Bit Packing 2/1, Display5/1
  In4/1 -> Bit Packing 4/1, Display7/1
  Cast To Double1/1 -> Double/1

== system openWaterModel/Sensor Processing/IMU Processing/Kite Measurements /binary2double11 ==
  In1 : Inport
  In2 : Inport  Port=2
  In3 : Inport  Port=3
  In4 : Inport  Port=4
  Bit Packing {,1..4} (5 alike) : xpcutilitieslib/Bit Packing 
      settings: SourceProductBaseCode=XP
  Bit Shift1 : hdlsllib/Logic and Bit Operations/Bit Shift  mode=Shift Left Logical  N=16
  Bit Shift2 : hdlsllib/Logic and Bit Operations/Bit Shift  mode=Shift Left Logical  N=24
  Bit Shift3 : hdlsllib/Logic and Bit Operations/Bit Shift  mode=Shift Left Logical  N=8
  Bitwise Operator : simulink/Logic and Bit Operations/Bitwise Operator  logicop=OR  UseBitMask=off  NumInputPorts=4  BitMask=bin2dec('00000000')  BitMaskRealWorld=Stored Integer
  Cast To Double1 : DataTypeConversion  OutDataTypeStr=double
  Display{3,5..7,10..14} (9 alike) : Display
      settings: Format=hex (Stored Integer)
  Double : Outport
  wires:
  Bit Shift1/1 -> Bitwise Operator/2, Display10/1
  Bitwise Operator/1 -> Display14/1, "Bit Packing "/1
  Bit Packing 1/1 -> Bit Shift2/1
  Bit Packing 4/1 -> Bitwise Operator/4, Display13/1
  In1/1 -> Bit Packing 1/1, Display3/1
  In3/1 -> Bit Packing 3/1, Display6/1
  Bit Shift2/1 -> Bitwise Operator/1, Display11/1
  Bit Packing 2/1 -> Bit Shift1/1
  "Bit Packing "/1 -> Cast To Double1/1
  Bit Shift3/1 -> Bitwise Operator/3, Display12/1
  Bit Packing 3/1 -> Bit Shift3/1
  In2/1 -> Bit Packing 2/1, Display5/1
  In4/1 -> Bit Packing 4/1, Display7/1
  Cast To Double1/1 -> Double/1

== system openWaterModel/Sensor Processing/IMU Processing/Kite Measurements /binary2double12 ==
  In1 : Inport
  In2 : Inport  Port=2
  In3 : Inport  Port=3
  In4 : Inport  Port=4
  Bit Packing {,1..4} (5 alike) : xpcutilitieslib/Bit Packing 
      settings: SourceProductBaseCode=XP
  Bit Shift1 : hdlsllib/Logic and Bit Operations/Bit Shift  mode=Shift Left Logical  N=16
  Bit Shift2 : hdlsllib/Logic and Bit Operations/Bit Shift  mode=Shift Left Logical  N=24
  Bit Shift3 : hdlsllib/Logic and Bit Operations/Bit Shift  mode=Shift Left Logical  N=8
  Bitwise Operator : simulink/Logic and Bit Operations/Bitwise Operator  logicop=OR  UseBitMask=off  NumInputPorts=4  BitMask=bin2dec('00000000')  BitMaskRealWorld=Stored Integer
  Cast To Double1 : DataTypeConversion  OutDataTypeStr=double
  Display{3,5..7,10..14} (9 alike) : Display
      settings: Format=hex (Stored Integer)
  Double : Outport
  wires:
  Bit Shift1/1 -> Bitwise Operator/2, Display10/1
  Bitwise Operator/1 -> Display14/1, "Bit Packing "/1
  Bit Packing 1/1 -> Bit Shift2/1
  Bit Packing 4/1 -> Bitwise Operator/4, Display13/1
  In1/1 -> Bit Packing 1/1, Display3/1
  In3/1 -> Bit Packing 3/1, Display6/1
  Bit Shift2/1 -> Bitwise Operator/1, Display11/1
  Bit Packing 2/1 -> Bit Shift1/1
  "Bit Packing "/1 -> Cast To Double1/1
  Bit Shift3/1 -> Bitwise Operator/3, Display12/1
  Bit Packing 3/1 -> Bit Shift3/1
  In2/1 -> Bit Packing 2/1, Display5/1
  In4/1 -> Bit Packing 4/1, Display7/1
  Cast To Double1/1 -> Double/1

== system openWaterModel/Sensor Processing/IMU Processing/Kite Measurements /binary2double13 ==
  In1 : Inport
  In2 : Inport  Port=2
  In3 : Inport  Port=3
  In4 : Inport  Port=4
  Bit Packing {,1..4} (5 alike) : xpcutilitieslib/Bit Packing 
      settings: SourceProductBaseCode=XP
  Bit Shift1 : hdlsllib/Logic and Bit Operations/Bit Shift  mode=Shift Left Logical  N=16
  Bit Shift2 : hdlsllib/Logic and Bit Operations/Bit Shift  mode=Shift Left Logical  N=24
  Bit Shift3 : hdlsllib/Logic and Bit Operations/Bit Shift  mode=Shift Left Logical  N=8
  Bitwise Operator : simulink/Logic and Bit Operations/Bitwise Operator  logicop=OR  UseBitMask=off  NumInputPorts=4  BitMask=bin2dec('00000000')  BitMaskRealWorld=Stored Integer
  Cast To Double1 : DataTypeConversion  OutDataTypeStr=double
  Display{3,5..7,10..14} (9 alike) : Display
      settings: Format=hex (Stored Integer)
  Double : Outport
  wires:
  Bit Shift1/1 -> Bitwise Operator/2, Display10/1
  Bitwise Operator/1 -> Display14/1, "Bit Packing "/1
  Bit Packing 1/1 -> Bit Shift2/1
  Bit Packing 4/1 -> Bitwise Operator/4, Display13/1
  In1/1 -> Bit Packing 1/1, Display3/1
  In3/1 -> Bit Packing 3/1, Display6/1
  Bit Shift2/1 -> Bitwise Operator/1, Display11/1
  Bit Packing 2/1 -> Bit Shift1/1
  "Bit Packing "/1 -> Cast To Double1/1
  Bit Shift3/1 -> Bitwise Operator/3, Display12/1
  Bit Packing 3/1 -> Bit Shift3/1
  In2/1 -> Bit Packing 2/1, Display5/1
  In4/1 -> Bit Packing 4/1, Display7/1
  Cast To Double1/1 -> Double/1

== system openWaterModel/Sensor Processing/IMU Processing/Kite Measurements /binary2double14 ==
  In1 : Inport
  In2 : Inport  Port=2
  In3 : Inport  Port=3
  In4 : Inport  Port=4
  Bit Packing {,1..4} (5 alike) : xpcutilitieslib/Bit Packing 
      settings: SourceProductBaseCode=XP
  Bit Shift1 : hdlsllib/Logic and Bit Operations/Bit Shift  mode=Shift Left Logical  N=16
  Bit Shift2 : hdlsllib/Logic and Bit Operations/Bit Shift  mode=Shift Left Logical  N=24
  Bit Shift3 : hdlsllib/Logic and Bit Operations/Bit Shift  mode=Shift Left Logical  N=8
  Bitwise Operator : simulink/Logic and Bit Operations/Bitwise Operator  logicop=OR  UseBitMask=off  NumInputPorts=4  BitMask=bin2dec('00000000')  BitMaskRealWorld=Stored Integer
  Cast To Double1 : DataTypeConversion  OutDataTypeStr=double
  Display{3,5..7,10..14} (9 alike) : Display
      settings: Format=hex (Stored Integer)
  Double : Outport
  wires:
  Bit Shift1/1 -> Bitwise Operator/2, Display10/1
  Bitwise Operator/1 -> Display14/1, "Bit Packing "/1
  Bit Packing 1/1 -> Bit Shift2/1
  Bit Packing 4/1 -> Bitwise Operator/4, Display13/1
  In1/1 -> Bit Packing 1/1, Display3/1
  In3/1 -> Bit Packing 3/1, Display6/1
  Bit Shift2/1 -> Bitwise Operator/1, Display11/1
  Bit Packing 2/1 -> Bit Shift1/1
  "Bit Packing "/1 -> Cast To Double1/1
  Bit Shift3/1 -> Bitwise Operator/3, Display12/1
  Bit Packing 3/1 -> Bit Shift3/1
  In2/1 -> Bit Packing 2/1, Display5/1
  In4/1 -> Bit Packing 4/1, Display7/1
  Cast To Double1/1 -> Double/1

== system openWaterModel/Sensor Processing/IMU Processing/Kite Measurements /binary2double15 ==
  In1 : Inport
  In2 : Inport  Port=2
  In3 : Inport  Port=3
  In4 : Inport  Port=4
  Bit Packing {,1..4} (5 alike) : xpcutilitieslib/Bit Packing 
      settings: SourceProductBaseCode=XP
  Bit Shift1 : hdlsllib/Logic and Bit Operations/Bit Shift  mode=Shift Left Logical  N=16
  Bit Shift2 : hdlsllib/Logic and Bit Operations/Bit Shift  mode=Shift Left Logical  N=24
  Bit Shift3 : hdlsllib/Logic and Bit Operations/Bit Shift  mode=Shift Left Logical  N=8
  Bitwise Operator : simulink/Logic and Bit Operations/Bitwise Operator  logicop=OR  UseBitMask=off  NumInputPorts=4  BitMask=bin2dec('00000000')  BitMaskRealWorld=Stored Integer
  Cast To Double1 : DataTypeConversion  OutDataTypeStr=double
  Display{3,5..7,10..14} (9 alike) : Display
      settings: Format=hex (Stored Integer)
  Double : Outport
  wires:
  Bit Shift1/1 -> Bitwise Operator/2, Display10/1
  Bitwise Operator/1 -> Display14/1, "Bit Packing "/1
  Bit Packing 1/1 -> Bit Shift2/1
  Bit Packing 4/1 -> Bitwise Operator/4, Display13/1
  In1/1 -> Bit Packing 1/1, Display3/1
  In3/1 -> Bit Packing 3/1, Display6/1
  Bit Shift2/1 -> Bitwise Operator/1, Display11/1
  Bit Packing 2/1 -> Bit Shift1/1
  "Bit Packing "/1 -> Cast To Double1/1
  Bit Shift3/1 -> Bitwise Operator/3, Display12/1
  Bit Packing 3/1 -> Bit Shift3/1
  In2/1 -> Bit Packing 2/1, Display5/1
  In4/1 -> Bit Packing 4/1, Display7/1
  Cast To Double1/1 -> Double/1

== system openWaterModel/Sensor Processing/IMU Processing/Kite Measurements /binary2double16 ==
  In1 : Inport
  In2 : Inport  Port=2
  In3 : Inport  Port=3
  In4 : Inport  Port=4
  Bit Packing {,1..4} (5 alike) : xpcutilitieslib/Bit Packing 
      settings: SourceProductBaseCode=XP
  Bit Shift1 : hdlsllib/Logic and Bit Operations/Bit Shift  mode=Shift Left Logical  N=16
  Bit Shift2 : hdlsllib/Logic and Bit Operations/Bit Shift  mode=Shift Left Logical  N=24
  Bit Shift3 : hdlsllib/Logic and Bit Operations/Bit Shift  mode=Shift Left Logical  N=8
  Bitwise Operator : simulink/Logic and Bit Operations/Bitwise Operator  logicop=OR  UseBitMask=off  NumInputPorts=4  BitMask=bin2dec('00000000')  BitMaskRealWorld=Stored Integer
  Cast To Double1 : DataTypeConversion  OutDataTypeStr=double
  Display{3,5..7,10..14} (9 alike) : Display
      settings: Format=hex (Stored Integer)
  Double : Outport
  wires:
  Bit Shift1/1 -> Bitwise Operator/2, Display10/1
  Bitwise Operator/1 -> Display14/1, "Bit Packing "/1
  Bit Packing 1/1 -> Bit Shift2/1
  Bit Packing 4/1 -> Bitwise Operator/4, Display13/1
  In1/1 -> Bit Packing 1/1, Display3/1
  In3/1 -> Bit Packing 3/1, Display6/1
  Bit Shift2/1 -> Bitwise Operator/1, Display11/1
  Bit Packing 2/1 -> Bit Shift1/1
  "Bit Packing "/1 -> Cast To Double1/1
  Bit Shift3/1 -> Bitwise Operator/3, Display12/1
  Bit Packing 3/1 -> Bit Shift3/1
  In2/1 -> Bit Packing 2/1, Display5/1
  In4/1 -> Bit Packing 4/1, Display7/1
  Cast To Double1/1 -> Double/1

== system openWaterModel/Sensor Processing/IMU Processing/Kite Measurements /binary2double17 ==
  In1 : Inport
  In2 : Inport  Port=2
  In3 : Inport  Port=3
  In4 : Inport  Port=4
  Bit Packing {,1..4} (5 alike) : xpcutilitieslib/Bit Packing 
      settings: SourceProductBaseCode=XP
  Bit Shift1 : hdlsllib/Logic and Bit Operations/Bit Shift  mode=Shift Left Logical  N=16
  Bit Shift2 : hdlsllib/Logic and Bit Operations/Bit Shift  mode=Shift Left Logical  N=24
  Bit Shift3 : hdlsllib/Logic and Bit Operations/Bit Shift  mode=Shift Left Logical  N=8
  Bitwise Operator : simulink/Logic and Bit Operations/Bitwise Operator  logicop=OR  UseBitMask=off  NumInputPorts=4  BitMask=bin2dec('00000000')  BitMaskRealWorld=Stored Integer
  Cast To Double1 : DataTypeConversion  OutDataTypeStr=double
  Display{3,5..7,10..14} (9 alike) : Display
      settings: Format=hex (Stored Integer)
  Double : Outport
  wires:
  Cast To Double1/1 -> Double/1
  In4/1 -> Display7/1, Bit Packing 4/1
  In2/1 -> Display5/1, Bit Packing 2/1
  Bit Packing 3/1 -> Bit Shift3/1
  Bit Shift3/1 -> Display12/1, Bitwise Operator/3
  "Bit Packing "/1 -> Cast To Double1/1
  Bit Packing 2/1 -> Bit Shift1/1
  Bit Shift2/1 -> Display11/1, Bitwise Operator/1
  In3/1 -> Display6/1, Bit Packing 3/1
  In1/1 -> Display3/1, Bit Packing 1/1
  Bit Packing 4/1 -> Display13/1, Bitwise Operator/4
  Bit Packing 1/1 -> Bit Shift2/1
  Bitwise Operator/1 -> "Bit Packing "/1, Display14/1
  Bit Shift1/1 -> Display10/1, Bitwise Operator/2

== system openWaterModel/Sensor Processing/IMU Processing/Kite Measurements /binary2double18 ==
  In1 : Inport
  In2 : Inport  Port=2
  In3 : Inport  Port=3
  In4 : Inport  Port=4
  Bit Packing {,1..4} (5 alike) : xpcutilitieslib/Bit Packing 
      settings: SourceProductBaseCode=XP
  Bit Shift1 : hdlsllib/Logic and Bit Operations/Bit Shift  mode=Shift Left Logical  N=16
  Bit Shift2 : hdlsllib/Logic and Bit Operations/Bit Shift  mode=Shift Left Logical  N=24
  Bit Shift3 : hdlsllib/Logic and Bit Operations/Bit Shift  mode=Shift Left Logical  N=8
  Bitwise Operator : simulink/Logic and Bit Operations/Bitwise Operator  logicop=OR  UseBitMask=off  NumInputPorts=4  BitMask=bin2dec('00000000')  BitMaskRealWorld=Stored Integer
  Cast To Double1 : DataTypeConversion  OutDataTypeStr=double
  Display{3,5..7,10..14} (9 alike) : Display
      settings: Format=hex (Stored Integer)
  Double : Outport
  wires:
  Bit Shift1/1 -> Bitwise Operator/2, Display10/1
  Bitwise Operator/1 -> Display14/1, "Bit Packing "/1
  Bit Packing 1/1 -> Bit Shift2/1
  Bit Packing 4/1 -> Bitwise Operator/4, Display13/1
  In1/1 -> Bit Packing 1/1, Display3/1
  In3/1 -> Bit Packing 3/1, Display6/1
  Bit Shift2/1 -> Bitwise Operator/1, Display11/1
  Bit Packing 2/1 -> Bit Shift1/1
  "Bit Packing "/1 -> Cast To Double1/1
  Bit Shift3/1 -> Bitwise Operator/3, Display12/1
  Bit Packing 3/1 -> Bit Shift3/1
  In2/1 -> Bit Packing 2/1, Display5/1
  In4/1 -> Bit Packing 4/1, Display7/1
  Cast To Double1/1 -> Double/1

== system openWaterModel/Sensor Processing/IMU Processing/Kite Measurements /binary2double19 ==
  In1 : Inport
  In2 : Inport  Port=2
  In3 : Inport  Port=3
  In4 : Inport  Port=4
  Bit Packing {,1..4} (5 alike) : xpcutilitieslib/Bit Packing 
      settings: SourceProductBaseCode=XP
  Bit Shift1 : hdlsllib/Logic and Bit Operations/Bit Shift  mode=Shift Left Logical  N=16
  Bit Shift2 : hdlsllib/Logic and Bit Operations/Bit Shift  mode=Shift Left Logical  N=24
  Bit Shift3 : hdlsllib/Logic and Bit Operations/Bit Shift  mode=Shift Left Logical  N=8
  Bitwise Operator : simulink/Logic and Bit Operations/Bitwise Operator  logicop=OR  UseBitMask=off  NumInputPorts=4  BitMask=bin2dec('00000000')  BitMaskRealWorld=Stored Integer
  Cast To Double1 : DataTypeConversion  OutDataTypeStr=double
  Display{3,5..7,10..14} (9 alike) : Display
      settings: Format=hex (Stored Integer)
  Double : Outport
  wires:
  Cast To Double1/1 -> Double/1
  In4/1 -> Display7/1, Bit Packing 4/1
  In2/1 -> Display5/1, Bit Packing 2/1
  Bit Packing 3/1 -> Bit Shift3/1
  Bit Shift3/1 -> Display12/1, Bitwise Operator/3
  "Bit Packing "/1 -> Cast To Double1/1
  Bit Packing 2/1 -> Bit Shift1/1
  Bit Shift2/1 -> Display11/1, Bitwise Operator/1
  In3/1 -> Display6/1, Bit Packing 3/1
  In1/1 -> Display3/1, Bit Packing 1/1
  Bit Packing 4/1 -> Display13/1, Bitwise Operator/4
  Bit Packing 1/1 -> Bit Shift2/1
  Bitwise Operator/1 -> "Bit Packing "/1, Display14/1
  Bit Shift1/1 -> Display10/1, Bitwise Operator/2

== system openWaterModel/Sensor Processing/IMU Processing/Kite Measurements /binary2double2 ==
  In1 : Inport
  In2 : Inport  Port=2
  In3 : Inport  Port=3
  In4 : Inport  Port=4
  Bit Packing {,1..4} (5 alike) : xpcutilitieslib/Bit Packing 
      settings: SourceProductBaseCode=XP
  Bit Shift1 : hdlsllib/Logic and Bit Operations/Bit Shift  mode=Shift Left Logical  N=16
  Bit Shift2 : hdlsllib/Logic and Bit Operations/Bit Shift  mode=Shift Left Logical  N=24
  Bit Shift3 : hdlsllib/Logic and Bit Operations/Bit Shift  mode=Shift Left Logical  N=8
  Bitwise Operator : simulink/Logic and Bit Operations/Bitwise Operator  logicop=OR  UseBitMask=off  NumInputPorts=4  BitMask=bin2dec('00000000')  BitMaskRealWorld=Stored Integer
  Cast To Double1 : DataTypeConversion  OutDataTypeStr=double
  Display{3,5..7,10..14} (9 alike) : Display
      settings: Format=hex (Stored Integer)
  Double : Outport
  wires:
  Bit Shift1/1 -> Bitwise Operator/2, Display10/1
  Bitwise Operator/1 -> Display14/1, "Bit Packing "/1
  Bit Packing 1/1 -> Bit Shift2/1
  Bit Packing 4/1 -> Bitwise Operator/4, Display13/1
  In1/1 -> Bit Packing 1/1, Display3/1
  In3/1 -> Bit Packing 3/1, Display6/1
  Bit Shift2/1 -> Bitwise Operator/1, Display11/1
  Bit Packing 2/1 -> Bit Shift1/1
  "Bit Packing "/1 -> Cast To Double1/1
  Bit Shift3/1 -> Bitwise Operator/3, Display12/1
  Bit Packing 3/1 -> Bit Shift3/1
  In2/1 -> Bit Packing 2/1, Display5/1
  In4/1 -> Bit Packing 4/1, Display7/1
  Cast To Double1/1 -> Double/1
